simulink model "Motor"  (R2022a)
settings: Solver=VariableStepAuto  StartTime=0.0  StopTime=2  MaxStep=1e-4  RelTol=1e-3
InitFcn:
  | Rs=1.405
  | Rr=1.395
  | Ls=0.178039
  | Lm=0.1722
  | Lr=0.178039
  | J=0.0131
  | P=4
  | w=2*pi*50
  | Tl=26.50
libraries: spsdq0toabcLib x1, spsabctodq0Lib x1
settings Model: Creator=Deepak  LastModifiedBy=Asus X513
settings SolverCC: AlgebraicLoopSolver=TrustRegion
settings DebuggingCC: UnconnectedInputMsg=warning  UnconnectedOutputMsg=warning  UnconnectedLineMsg=warning  SFMachineParentedDataDiag=warning
settings SFSimCC: CustomCodeUndefinedFunction=UseInterfaceOnly

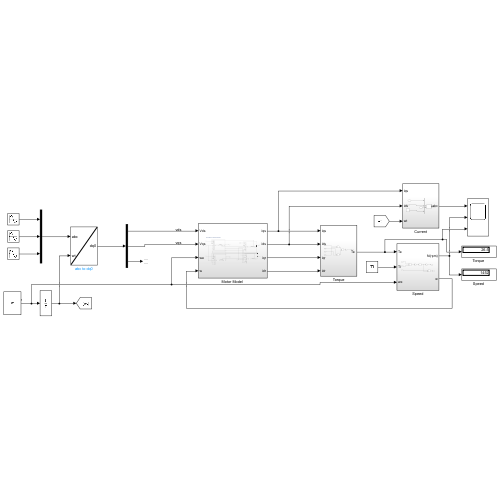
[thumbnail: Simulink's stored preview of the top-level diagram]
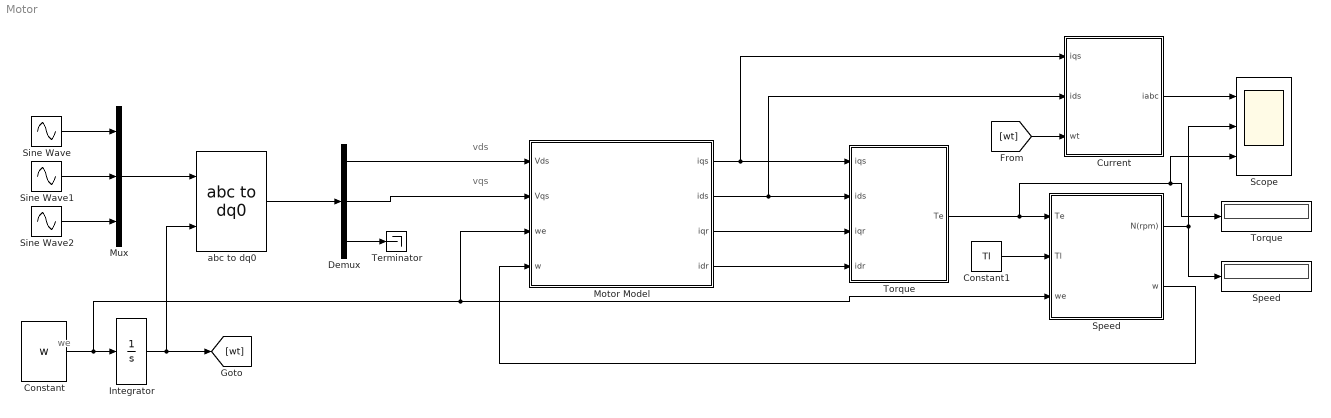
== system Motor ==
  note: we
  note: vqs
  note: vds
  Constant : Constant  Value=w
  Constant1 : Constant  Value=Tl
  Current : Subsystem
  Demux : Demux  Outputs=3
  Integrator : Integrator
  "Motor Model " : Subsystem
  Mux : Mux  Inputs=3
  Scope : Scope  NumInputPorts=3
  Sine Wave : Sin  Amplitude=373.5  Frequency=w  SampleTime=0
  Sine Wave1 : Sin  Amplitude=373.5  Frequency=w  Phase=-(2*pi)/3  SampleTime=0
  Sine Wave2 : Sin  Amplitude=373.5  Frequency=w  Phase=(2*pi)/3  SampleTime=0
  Speed : Subsystem
  "Speed " : Display
  Terminator : Terminator
  Torque : Subsystem
  "Torque " : Display
  abc to dq0 : spsabctodq0Lib/abc to dq0  Alignment=90 degrees behind phase A axis
  wires:
  Sine Wave1/1 -> Mux/2
  Sine Wave/1 -> Mux/1
  Sine Wave2/1 -> Mux/3
  Mux/1 -> abc to dq0/1
  Constant/1 -> Speed/3(we), "Motor Model "/3(we), Integrator/1
  Integrator/1 -> [wt], abc to dq0/2
  abc to dq0/1 -> Demux/1
  Demux/3 -> Terminator/1
  Demux/1 -> "Motor Model "/1("Vds ")
  Demux/2 -> "Motor Model "/2("Vqs ")
  "Motor Model "/1(iqs) -> Torque/1(iqs), Current/1(iqs)
  "Motor Model "/2(ids) -> Torque/2(ids), Current/2(ids)
  "Motor Model "/3(iqr) -> Torque/3(iqr)
  "Motor Model "/4(idr) -> Torque/4(idr)
  Torque/1("Te ") -> Speed/1(Te), "Torque "/1, Scope/3
  Constant1/1 -> Speed/2(Tl)
  Speed/2(w) -> "Motor Model "/4(w)
  [wt] -> Current/3(wt)
  Current/1(iabc) -> Scope/1
  Speed/1(N(rpm)) -> "Speed "/1, Scope/2

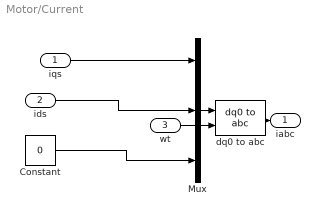
== system Motor/Current ==
  iqs : Inport
  ids : Inport  Port=2
  wt : Inport  Port=3
  Constant : Constant  Value=0
  Mux : Mux  Inputs=3
  dq0 to abc : spsdq0toabcLib/dq0 to abc  Alignment=90 degrees behind phase A axis
  iabc : Outport  VectorParamsAs1DForOutWhenUnconnected=off
  wires:
  Constant/1 -> Mux/3
  Mux/1 -> dq0 to abc/1
  ids/1 -> Mux/2
  iqs/1 -> Mux/1
  wt/1 -> dq0 to abc/2
  dq0 to abc/1 -> iabc/1

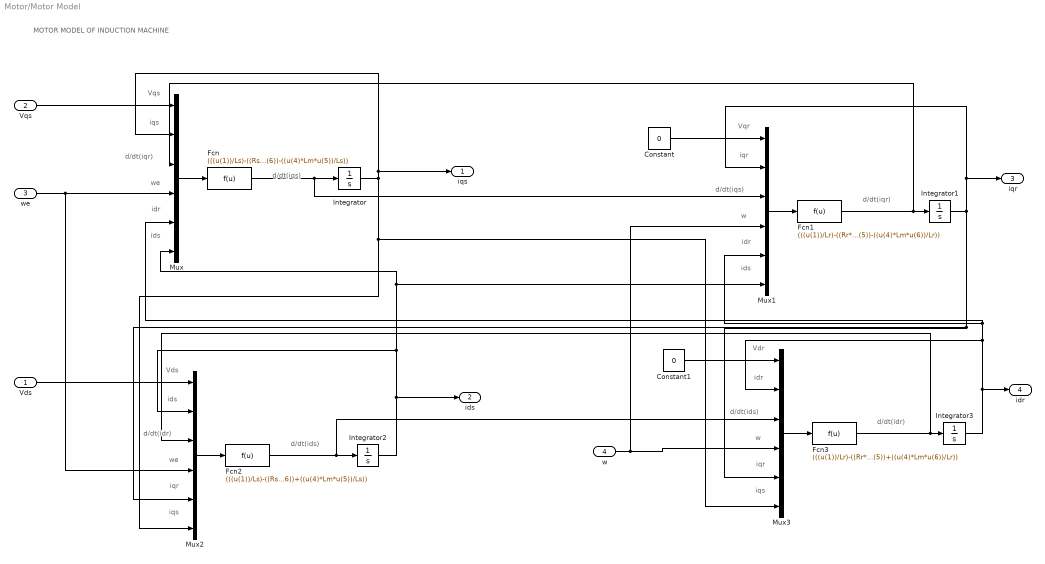
== system Motor/Motor Model  ==
  note: d/dt(iqs)
  note: ids
  note: idr
  note: we
  note: d/dt(iqr)
  note: iqs
  note: Vqs
  note: MOTOR MODEL OF INDUCTION MACHINE
  note: d/dt(iqr)
  note: ids
  note: d/dt(iqs)
  note: w
  note: idr
  note: Vqr
  note: iqr
  note: d/dt(ids)
  note: iqs
  note: d/dt(idr)
  note: we
  note: iqr
  note: Vds
  note: ids
  note: iqr
  note: w
  note: Vdr
  note: d/dt(ids)
  note: idr
  note: iqs
  note: d/dt(idr)
  "Vds " : Inport
  "Vqs " : Inport  Port=2
  we : Inport  Port=3
  w : Inport  Port=4
  Constant : Constant  Value=0
  Constant1 : Constant  Value=0
  Fcn : Fcn  Expr=(((u(1))/Ls)-((Rs*u(2))/Ls)-((u(3)*Lm)/Ls)-(u(4)*u(6))-((u(4)*Lm*u(5))/Ls))
  Fcn1 : Fcn  Expr=(((u(1))/Lr)-((Rr*u(2))/Lr)-((u(3)*Lm)/Lr)-(u(4)*u(5))-((u(4)*Lm*u(6))/Lr))
  Fcn2 : Fcn  Expr=(((u(1))/Ls)-((Rs*u(2))/Ls)-((u(3)*Lm)/Ls)+(u(4)*u(6))+((u(4)*Lm*u(5))/Ls))
  Fcn3 : Fcn  Expr=(((u(1))/Lr)-((Rr*u(2))/Lr)-((u(3)*Lm)/Lr)+(u(4)*u(5))+((u(4)*Lm*u(6))/Lr))
  Integrator{,1..3} (4 alike) : Integrator
  Mux{,1..3} (4 alike) : Mux  Inputs=6
  iqs : Outport  VectorParamsAs1DForOutWhenUnconnected=off
  ids : Outport  Port=2  VectorParamsAs1DForOutWhenUnconnected=off
  iqr : Outport  Port=3  VectorParamsAs1DForOutWhenUnconnected=off
  idr : Outport  Port=4  VectorParamsAs1DForOutWhenUnconnected=off
  wires:
  Integrator3/1 -> idr/1, Mux3/2, Mux1/5, Mux/5
  Mux/1 -> Fcn/1
  Fcn2/1 -> Mux3/3, Integrator2/1
  Integrator/1 -> iqs/1, Mux/2, Mux3/6, Mux2/6
  Integrator2/1 -> ids/1, Mux1/6, Mux/6, Mux2/2
  Integrator1/1 -> iqr/1, Mux1/2, Mux3/5, Mux2/5
  Constant/1 -> Mux1/1
  w/1 -> Mux1/4, Mux3/4
  "Vds "/1 -> Mux2/1
  Fcn3/1 -> Mux2/3, Integrator3/1
  Constant1/1 -> Mux3/1
  Fcn1/1 -> Mux/3, Integrator1/1
  "Vqs "/1 -> Mux/1
  Mux2/1 -> Fcn2/1
  Mux3/1 -> Fcn3/1
  we/1 -> Mux2/4, Mux/4
  Fcn/1 -> Mux1/3, Integrator/1
  Mux1/1 -> Fcn1/1

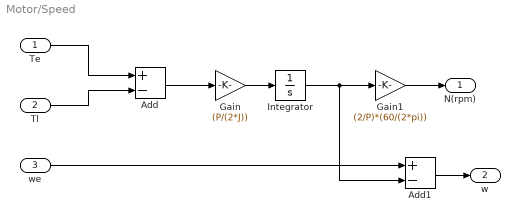
== system Motor/Speed ==
  Te : Inport
  Tl : Inport  Port=2
  we : Inport  Port=3
  Add : Sum  Inputs=+-
  Add1 : Sum  Inputs=+-
  Gain : Gain  Gain=(P/(2*J))
  Gain1 : Gain  Gain=(2/P)*(60/(2*pi))
  Integrator : Integrator
  N(rpm) : Outport  VectorParamsAs1DForOutWhenUnconnected=off
  w : Outport  Port=2  VectorParamsAs1DForOutWhenUnconnected=off
  wires:
  we/1 -> Add1/1
  Tl/1 -> Add/2
  Integrator/1 -> Add1/2, Gain1/1
  Te/1 -> Add/1
  Add/1 -> Gain/1
  Gain1/1 -> N(rpm)/1
  Gain/1 -> Integrator/1
  Add1/1 -> w/1

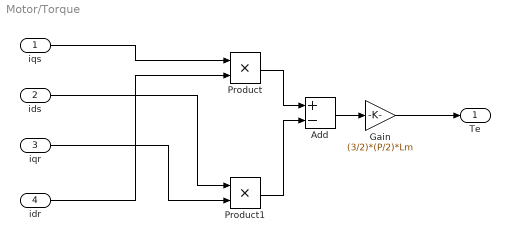
== system Motor/Torque ==
  iqs : Inport
  ids : Inport  Port=2
  iqr : Inport  Port=3
  idr : Inport  Port=4
  Add : Sum  Inputs=+-
  Gain : Gain  Gain=(3/2)*(P/2)*Lm
  Product : Product
  Product1 : Product
  "Te " : Outport  VectorParamsAs1DForOutWhenUnconnected=off
  wires:
  ids/1 -> Product1/1
  Product1/1 -> Add/2
  iqr/1 -> Product1/2
  idr/1 -> Product/2
  iqs/1 -> Product/1
  Gain/1 -> "Te "/1
  Add/1 -> Gain/1
  Product/1 -> Add/1
